simulink model "SFDC_Motor_for_Traction"  (R2020b)
settings: Solver=ode23s  StartTime=0.0  StopTime=800  EnableMultiTasking=on
values from neighbouring files (symbols this model uses):
  beta = P_trac/3/w_n^2    (= 0.976675486798)    [SFDC_Motor_for_Traction_data_script.m]
  En = eta*V_n    (= 540)    [SFDC_Motor_for_Traction_data_script.m]
  F1 = v_max/w_n    (= 0.0530785562633)    [SFDC_Motor_for_Traction_data_script.m]
  F3 = w_n/v_r    (= 5.23333333333)    [SFDC_Motor_for_Traction_data_script.m]
  Ie = 1    [SFDC_Motor_for_Traction_data_script.m]
  J = M*v_max^2/w_n^2    (= 73.2506615098)    [SFDC_Motor_for_Traction_data_script.m]
  K = T_n/(I_n*Ie)    (= 1.71974522293)    [SFDC_Motor_for_Traction_data_script.m]
  ki_ia = wc_ia*Ra    (= 16.8230769231)    [SFDC_Motor_for_Traction_data_script.m]
  ki_ie = wc_ie*Re    (= 2400)    [SFDC_Motor_for_Traction_data_script.m]
  ki_w = wc_w*beta    (= 0.976675486798)    [SFDC_Motor_for_Traction_data_script.m]
  kp_ia = wc_ia*La    (= 0.168230769231)    [SFDC_Motor_for_Traction_data_script.m]
  kp_ie = wc_ie*Le    (= 2400)    [SFDC_Motor_for_Traction_data_script.m]
  kp_w = wc_w*J    (= 73.2506615098)    [SFDC_Motor_for_Traction_data_script.m]
  La = Ra*tau_a    (= 0.000841153846154)    [SFDC_Motor_for_Traction_data_script.m]
  Le = Re*tau_e    (= 120)    [SFDC_Motor_for_Traction_data_script.m]
  M = m_t+m_p*n_p    (= 26000)    [SFDC_Motor_for_Traction_data_script.m]
  Ra = (P_el-P_tot)/I_n^2    (= 0.0841153846154)    [SFDC_Motor_for_Traction_data_script.m]
  Re = Ve/Ie    (= 120)    [SFDC_Motor_for_Traction_data_script.m]
  T_n = P_tot/w_n    (= 1226.70441142)    [SFDC_Motor_for_Traction_data_script.m]
  V_n = 600    [SFDC_Motor_for_Traction_data_script.m]
  Ve = 120    [SFDC_Motor_for_Traction_data_script.m]
settings Model: Creator=matti  LastModifiedBy=Gianciccetto
settings DataIOCC: LimitDataPoints=on  SaveFormat=Array  ReturnWorkspaceOutputs=off
settings OptimizationCC: LifeSpan=inf
settings DebuggingCC: SFUnexpectedBacktrackingDiag=warning  SFNoUnconditionalDefaultTransitionDiag=warning  SFExecutionAtInitializationDiag=none  ArithmeticOperatorsInVariantConditions=warning
settings HardwareCC: ProdBitPerPointer=32  ProdBitPerSizeT=32  ProdBitPerPtrDiffT=32  ProdLargestAtomicFloat=None  ProdIntDivRoundTo=Undefined  ProdEndianess=Unspecified  ProdWordSize=32  ProdHWDeviceType=32-bit Generic
settings ModelReferenceCC: PropagateSignalLabelsOutOfModel=off
settings SFSimCC: SimUseLocalCustomCode=off  CustomCodeUndefinedFunction=UseInterfaceOnly
settings RTWCC: RTWUseLocalCustomCode=off
settings CodeAppCC: StateflowObjectComments=on
settings GRTTargetCC: TargetLangStandard=C89/C90 (ANSI)
settings ConfigComp: CovMetricSettings=dw  CovSaveCumulativeToWorkspaceVar=on  CovSaveSingleToWorkspaceVar=on  CovExternalEMLEnable=off  CovSFcnEnable=off

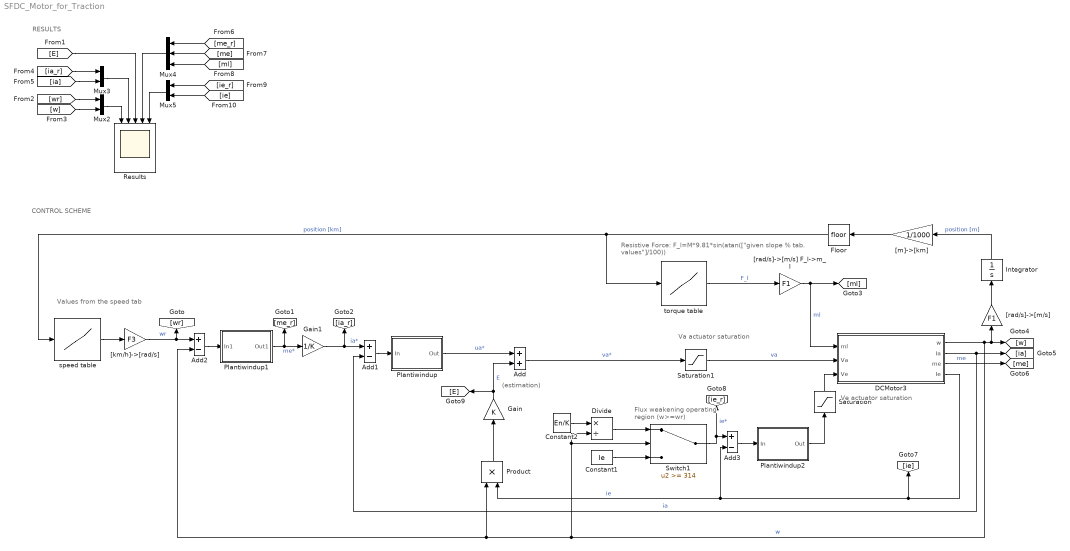
== system SFDC_Motor_for_Traction ==
  note: CONTROL SCHEME
  note: RESULTS
  note: Flux weakening
      | operating region (w>=wr)
  note: Values from
      | the speed tab
  note: (estimation)
  note: Ve actuator
      |  saturation
  note: Va actuator
      |  saturation
  note: Resistive Force:
      |  F_l=M*9.81*sin(atan(["given slope % tab. values"]/100))
  Add : Sum
  Add1 : Sum  Inputs=+-
  Add2 : Sum  Inputs=+-
  Add3 : Sum  Inputs=+-
  Constant1 : Constant  Value=Ie
  Constant2 : Constant  Value=En/K
  DCMotor3 : Subsystem
      mask Display:
      | disp('DC motor\nseparately-excited')
      | port_label('input', 1, 'ml')
      | port_label('input', 2, 'va')
      | port_label('input', 3, 've')
      | port_label('output', 1, 'omega')
      | port_label('output', 2, 'ia')
      | port_label('output', 3, 'me')
      | port_label('output', 4, 'ie')
  Divide : Product  Inputs=*/
  Floor : Rounding
  Gain : Gain  Gain=K
  Gain1 : Gain  Gain=1/K
  Integrator : Integrator
  Mux2 : Mux  Inputs=2
  Mux3 : Mux  Inputs=2
  Mux4 : Mux  Inputs=3
  Mux5 : Mux  Inputs=2
  PIantiwindup : Subsystem  mask{Kp=kp_ia, Ki=ki_ia, sat_up=V_n-En, sat_down=-(V_n-En)}
      mask prompts: sat_up "Upper sat. limit"; sat_down "Lower Sat. Limit"
      mask Display: disp('armature\ncurrent\ncontroller\n(PI)')
  PIantiwindup1 : Subsystem  mask{Kp=kp_w, Ki=ki_w, sat_up=T_n, sat_down=-T_n}
      mask prompts: sat_up "Upper sat. limit"; sat_down "Lower Sat. Limit"
      mask Display: disp('speed\ncontroller\n(PI)')
  PIantiwindup2 : Subsystem  mask{Kp=kp_ie, Ki=ki_ie, sat_up=Ve, sat_down=-Ve}
      mask prompts: sat_up "Upper sat. limit"; sat_down "Lower Sat. Limit"
      mask Display: disp('excitation\ncurrent\ncontroller\n(PI)')
  Product : Product
  Results : Scope  NumInputPorts=5
  Saturation : Saturate  UpperLimit=120  LowerLimit=-120
  Saturation1 : Saturate  UpperLimit=600  LowerLimit=-600
  Switch1 : Switch  Threshold=314
  "[km/h]->[rad/s]" : Gain  Gain=F3
  "[m]->[km]" : Gain  Gain=1/1000
  "[rad/s]->[m/s]" : Gain  Gain=F1
  "[rad/s]->[m/s] F_l->m_l" : Gain  Gain=F1
  speed table : Lookup_n-D  NumberOfTableDimensions=1  BreakpointsForDimension1=[0 1 3 4 6 8 9 10]  Table=[35 60 60 75 60 60 35 0]  InterpMethod=Flat  InternalRulePriority=Speed  RndMeth=Simplest  InputSameDT=on
  torque table : Lookup_n-D  NumberOfTableDimensions=1  BreakpointsForDimension1=[0 1 3 4 6 8 9 10]  Table=M*9.81*sin(atan([0 0 0.05 0 0 -0.05 0 0]))  InterpMethod=Flat  InternalRulePriority=Speed  RndMeth=Simplest  InputSameDT=on
  wires:
  PIantiwindup/1(Out) -> Add/1  "ua*"
  Add1/1 -> PIantiwindup/1(In)
  PIantiwindup1/1(Out1) -> Gain1/1, [me_r]  "me*"
  "[km/h]->[rad/s]"/1 -> Add2/1, [wr]  "wr"
  Add2/1 -> PIantiwindup1/1(In1)
  Gain/1 -> [E], Add/2  "E"
  Gain1/1 -> Add1/1, [ia_r]  "ia*"
  speed table/1 -> "[km/h]->[rad/s]"/1
  Product/1 -> Gain/1
  "[rad/s]->[m/s] F_l->m_l"/1 -> DCMotor3/1(ml), [ml]  "ml"
  torque table/1 -> "[rad/s]->[m/s] F_l->m_l"/1  "F_l"
  Add3/1 -> PIantiwindup2/1(In)
  Switch1/1 -> [ie_r], Add3/1  "ie*"
  Constant1/1 -> Switch1/3
  Divide/1 -> Switch1/1
  Constant2/1 -> Divide/1
  DCMotor3/1(w) -> [w], "[rad/s]->[m/s]"/1, Divide/2, Switch1/2, Product/1, Add2/2  "w"
  "[rad/s]->[m/s]"/1 -> Integrator/1
  Integrator/1 -> "[m]->[km]"/1  "position [m]"
  "[m]->[km]"/1 -> Floor/1
  Floor/1 -> torque table/1, speed table/1  "position [km]"
  DCMotor3/2(Ia) -> Add1/2, [ia]  "ia"
  DCMotor3/3(me) -> [me]  "me"
  DCMotor3/4(Ie) -> [ie], Add3/2, Product/2  "ie"
  [wr] -> Mux2/1
  [w] -> Mux2/2
  Mux2/1 -> Results/1
  Mux5/1 -> Results/5
  Mux4/1 -> Results/4
  Mux3/1 -> Results/2
  [me_r] -> Mux4/1
  [me] -> Mux4/2
  [ml] -> Mux4/3
  [ie_r] -> Mux5/1
  [ie] -> Mux5/2
  [ia_r] -> Mux3/1
  [ia] -> Mux3/2
  Add/1 -> Saturation1/1  "va*"
  PIantiwindup2/1(Out) -> Saturation/1
  Saturation/1 -> DCMotor3/3(Ve)
  Saturation1/1 -> DCMotor3/2(Va)  "va"
  [E] -> Results/3

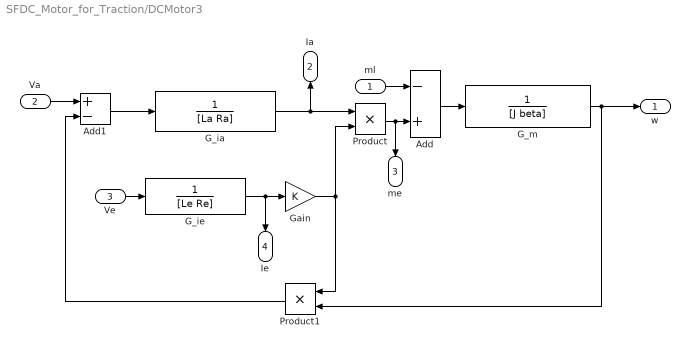
== system SFDC_Motor_for_Traction/DCMotor3 ==
  ml : Inport
  Va : Inport  Port=2
  Ve : Inport  Port=3
  Add : Sum  Inputs=-+
  Add1 : Sum  Inputs=+-
  G_ia : TransferFcn  Denominator=[La Ra]
  G_ie : TransferFcn  Denominator=[Le Re]
  G_m : TransferFcn  Denominator=[J beta]
  Gain : Gain  Gain=K
  Product : Product
  Product1 : Product
  w : Outport  VectorParamsAs1DForOutWhenUnconnected=off
  Ia : Outport  Port=2  VectorParamsAs1DForOutWhenUnconnected=off
  me : Outport  Port=3  VectorParamsAs1DForOutWhenUnconnected=off
  Ie : Outport  Port=4  VectorParamsAs1DForOutWhenUnconnected=off
  wires:
  ml/1 -> Add/1
  Add/1 -> G_m/1
  Gain/1 -> Product1/1, Product/2
  G_m/1 -> w/1, Product1/2
  Product1/1 -> Add1/2
  Add1/1 -> G_ia/1
  G_ia/1 -> Ia/1, Product/1
  Product/1 -> me/1, Add/2
  Ve/1 -> G_ie/1
  Va/1 -> Add1/1
  G_ie/1 -> Ie/1, Gain/1

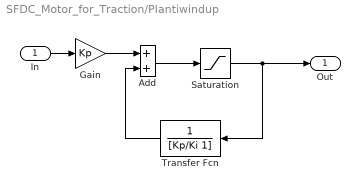
== system SFDC_Motor_for_Traction/PIantiwindup ==
  In : Inport
  Add : Sum
  Gain : Gain  Gain=Kp
  Saturation : Saturate  UpperLimit=sat_up  LowerLimit=sat_down
  Transfer Fcn : TransferFcn  Denominator=[Kp/Ki 1]
  Out : Outport  VectorParamsAs1DForOutWhenUnconnected=off
  wires:
  Saturation/1 -> Out/1, Transfer Fcn/1
  In/1 -> Gain/1
  Gain/1 -> Add/1
  Add/1 -> Saturation/1
  Transfer Fcn/1 -> Add/2

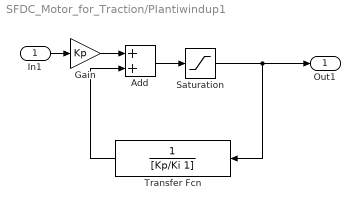
== system SFDC_Motor_for_Traction/PIantiwindup1 ==
  In1 : Inport
  Add : Sum
  Gain : Gain  Gain=Kp
  Saturation : Saturate  UpperLimit=sat_up  LowerLimit=sat_down
  Transfer Fcn : TransferFcn  Denominator=[Kp/Ki 1]
  Out1 : Outport  VectorParamsAs1DForOutWhenUnconnected=off
  wires:
  Transfer Fcn/1 -> Add/2
  Add/1 -> Saturation/1
  Gain/1 -> Add/1
  In1/1 -> Gain/1
  Saturation/1 -> Transfer Fcn/1, Out1/1

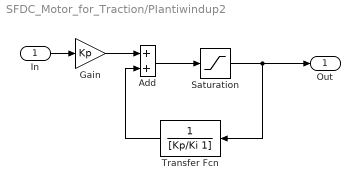
== system SFDC_Motor_for_Traction/PIantiwindup2 ==
  In : Inport
  Add : Sum
  Gain : Gain  Gain=Kp
  Saturation : Saturate  UpperLimit=sat_up  LowerLimit=sat_down
  Transfer Fcn : TransferFcn  Denominator=[Kp/Ki 1]
  Out : Outport  VectorParamsAs1DForOutWhenUnconnected=off
  wires:
  Saturation/1 -> Out/1, Transfer Fcn/1
  In/1 -> Gain/1
  Gain/1 -> Add/1
  Add/1 -> Saturation/1
  Transfer Fcn/1 -> Add/2
